simulink library "aerolibatmos2"  (Simulink 5.0)
values from neighbouring files (symbols this model uses):
  s = aeroliblist    [asbhelp.m]
undefined symbols (not defined in the file or in its folder): HDBK, kg, m, MIL, STD
libraries: aerolibconvert x7, aerolibatmos2 x3
settings Model: Creator=sgage  LastModifiedBy=sgage  ExtModeAutoUpdateStatusClock=off

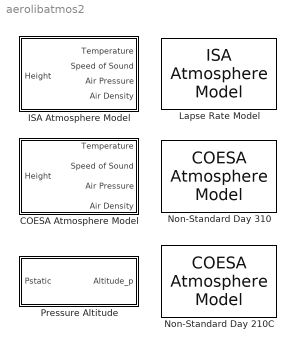
== system aerolibatmos2 ==
  COESA Atmosphere Model : Subsystem  mask(Atmosphere Model){units=Metric (MKS), spec=1976 COESA-extended U.S. Standard Atmosphere, model=Profile, profile_var=High temperature, profile_percent=1%, profile_alt=5 km (16404 ft), envelope_var=High temperature, envelope_percent=1%, action=Warning}
      mask prompts: spec "Specification:"; model "Atmospheric model type:"; profile_var "Extreme parameter:"; profile_percent "Frequency of occurrence:"; profile_alt "Altitude of extreme value:"; envelope_var "Extreme parameter:"; envelope_percent "Frequency of occurrence:"; action "Action for out of range input:"
      mask help:
      | Calculate various atmosphere models including 1976 COESA-extended U.S. Standard Atmosphere, MIL-HDBK-310, and MIL-STD-210C.  Given geopotential altitude, calculate absolute temperature, pressure and density using standard interpolation formulas.
      |
      | The COESA model extrapolates temperature linearly and pressure/density logarithmically beyond the range
      |
      | 	0 <= altitude <= 84852 meters (geopotential)
      |
      | The MIL specifications are not extrapolated beyond their defined altitudes which are typically
      |
      | 	0 <= altitude <= 80000 meters (geometric)
      |
      | Depending on the given information either density or pressure is calculated using a perfect gas relationship.
      |
      | The unit system selected applies to both input and outputs.
      mask init:
      | [ports] = aeroicon('aeroblkatmos','icon');
      | [x y miny txt] = aeroimage('atmosphere');
      mask Help: web(asbhelp('COESA Atmosphere Model'));
      mask StyleString: popup(Metric (MKS)|English (Velocity in ft/s)|English (Velocity in kts)),popup(1976 COESA-extended U.S. Standard Atmosphere|MIL-HDBK-310|MIL-STD-210C),popup(Profile|Envelope),popup(High temperature|Low temperature|High density|Low density),popup(1%|10%),popup(5 km (16404 ft)|10 km (32808 ft)|20 km (65617 ft)|30 km (98425 ft)|40 km (131234 ft)),popup(High temperature|Low temperature|High density|Low density|High pressure|Low pressure),popup(Extreme values|1%|5%|10%|20%),popup(None|Warning|Error)
      mask CallbackString: aeroicon('aeroblkatmos');|aeroicon('aeroblkatmos');|aeroicon('aeroblkatmos');||||||
      mask Display:
      | port_label(ports(1).type,ports(1).port,ports(1).txt,'texmode','on');
      | port_label(ports(2).type,ports(2).port,ports(2).txt,'texmode','on');
      | port_label(ports(3).type,ports(3).port,ports(3).txt,'texmode','on');
      | port_label(ports(4).type,ports(4).port,ports(4).txt,'texmode','on');
      | port_label(ports(5).type,ports(5).port,ports(5).txt,'texmode','on');
      | plot(x,y)
      | text(0.5,miny-.07,txt,'HorizontalAlignment','center');
  ISA Atmosphere Model : Subsystem  mask(International Standard Atmosphere Model){custom=off, g=9.80665, gamma=1.4, R=287.0531, L=0.0065, h_trop=11000, h_strat=20000, rho0=1.225, P0=101325, T0=288.15}
      mask prompts: custom "Change atmospheric parameters"; g "Acceleration due to gravity (m/s^2):"; gamma "Ratio of specific heats:"; R "Characteristic gas constant (J/Kg/K):"; L "Lapse rate (K/m):"; h_trop "Height of troposphere (m):"; h_strat "Height of tropopause (m):"; rho0 "Air density at mean sea level (Kg/m^3):"; P0 "Ambient pressure at mean sea level (N/m^2):"; T0 "Ambient temperature at mean sea level (K):"
      mask help:
      | Compute International Standard Atmosphere (ISA) model for altitudes between 0 Km and 20 Km using a lapse rate method.
      |
      | Select change atmospheric parameters to create custom atmosphere.
      mask init:
      | ports = aeroicon('aeroblkisa','icon');
      | [x y miny txt] = aeroimage('atmosphere');
      mask Help: web(asbhelp('isaatmospheremodel'));
      mask CallbackString: aeroicon('aeroblkisa')|||||||||
      mask Display:
      | port_label('input',1,'h (m)','texmode','on');
      | port_label('output',1,'T (K)','texmode','on');
      | port_label('output',2,'a (m/s)','texmode','on');
      | port_label('output',3,'P (Pa)','texmode','on');
      | port_label('output',4,'\rho (kg/m^3)','texmode','on');
      | plot(x,y)
      | text(0.5,miny-.07,txt,'HorizontalAlignment','center');
  Lapse Rate Model : aerolibatmos2/ISA Atmosphere Model  custom=on  g=9.80665  gamma=1.4  R=287.0531  L=0.0065  h_trop=11000  h_strat=20000  rho0=1.225  P0=101325  T0=288.15
  Non-Standard Day 210C : aerolibatmos2/COESA Atmosphere Model  units=Metric (MKS)  spec=MIL-STD-210C  model=Profile  profile_var=High temperature  profile_percent=1%  profile_alt=5 km (16404 ft)  envelope_var=High temperature  envelope_percent=1%  action=Warning
  Non-Standard Day 310 : aerolibatmos2/COESA Atmosphere Model  units=Metric (MKS)  spec=MIL-HDBK-310  model=Profile  profile_var=High temperature  profile_percent=1%  profile_alt=5 km (16404 ft)  envelope_var=High temperature  envelope_percent=1%  action=Warning
  Pressure Altitude : Subsystem  mask(Pressure Altitude){units=Metric (MKS), action=Warning}
      mask prompts: action "Action for out of range input:"
      mask help:
      | Calculate pressure altitude based on ambient pressure.
      |
      | Pressure altitude is the altitude in the 1976 COESA-extended U.S. Standard Atmosphere with specified ambient pressure.  Pressure altitude is also known as the mean sea level altitude (MSL).
      mask init:
      | ports = aeroicon('aeroblkpalt','icon');
      mask Help: web(asbhelp('pressurealtitude'));
      mask StyleString: popup(Metric (MKS)|English),popup(None|Warning|Error)
      mask Display:
      | port_label(ports(1).type,ports(1).port,ports(1).txt,'texmode','on');
      | port_label(ports(2).type,ports(2).port,ports(2).txt,'texmode','on');

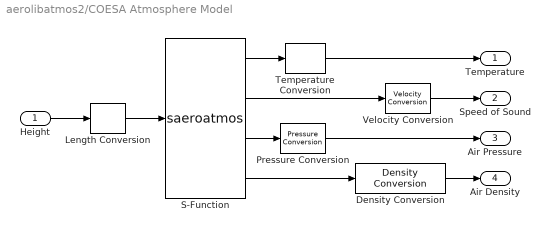
== system aerolibatmos2/COESA Atmosphere Model ==
  Height : Inport
  Density Conversion : aerolibconvert/Density Conversion  IU=kg/m^3  OU=kg/m^3
  Length Conversion : aerolibconvert/Length Conversion  IU=m  OU=m
  Pressure Conversion : aerolibconvert/Pressure Conversion  IU=Pa  OU=Pa
  S-Function : S-Function  FunctionName=saeroatmos  Parameters=spec,model,profile_var,profile_percent,profile_alt,envelope_var,envelope_percent,action  SFunctionModules=aeroatmcoesa aeroatmenvelope310 aeroatmenvelope210c aeroatmprofile310 aeroatmprofile210c
  Temperature Conversion : aerolibconvert/Temperature Conversion  IU=K  OU=K
  Velocity Conversion : aerolibconvert/Velocity Conversion  IU=m/s  OU=m/s
  Temperature : Outport
  Speed of Sound : Outport  Port=2
  Air Pressure : Outport  Port=3
  Air Density : Outport  Port=4
  wires:
  Length Conversion/1 -> S-Function/1
  Velocity Conversion/1 -> Speed of Sound/1
  S-Function/2 -> Velocity Conversion/1
  S-Function/1 -> Temperature Conversion/1
  S-Function/3 -> Pressure Conversion/1
  S-Function/4 -> Density Conversion/1
  Temperature Conversion/1 -> Temperature/1
  Height/1 -> Length Conversion/1
  Pressure Conversion/1 -> Air Pressure/1
  Density Conversion/1 -> Air Density/1

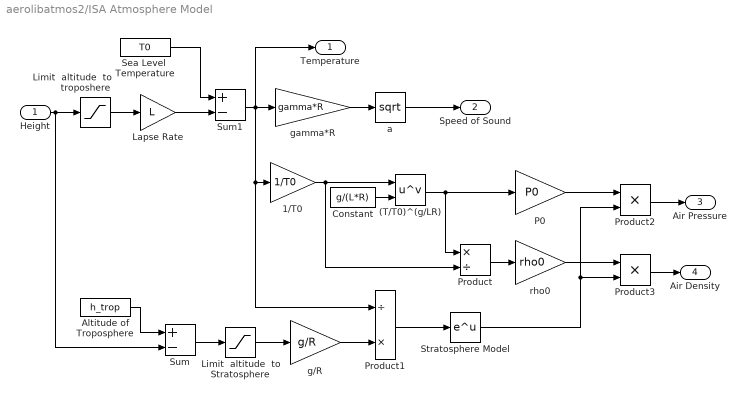
== system aerolibatmos2/ISA Atmosphere Model ==
  Height : Inport
  "(T/T0)^(g/LR) " : Math  Operator=pow
  1/T0 : Gain  Gain=1/T0  SaturateOnIntegerOverflow=on
  Altitude of Troposphere : Constant  Value=h_trop  ShowAdditionalParam=on
  Constant : Constant  Value=g/(L*R)  ShowAdditionalParam=on
  Lapse Rate : Gain  Gain=L  SaturateOnIntegerOverflow=on
  Limit  altitude  to Stratosphere : Saturate  UpperLimit=0  LowerLimit=h_trop-h_strat
  Limit  altitude  to troposhere : Saturate  UpperLimit=h_trop  LowerLimit=0
  P0 : Gain  Gain=P0  SaturateOnIntegerOverflow=on
  Product : Product  Inputs=*/  SaturateOnIntegerOverflow=on  InputSameDT=on
  Product1 : Product  Inputs=/*  SaturateOnIntegerOverflow=on  InputSameDT=on
  Product2 : Product  SaturateOnIntegerOverflow=on  InputSameDT=on
  Product3 : Product  SaturateOnIntegerOverflow=on  InputSameDT=on
  Sea Level  Temperature : Constant  Value=T0  ShowAdditionalParam=on
  Stratosphere Model : Math
  Sum : Sum  Inputs=+-  SaturateOnIntegerOverflow=on  InputSameDT=on
  Sum1 : Sum  Inputs=+-  SaturateOnIntegerOverflow=on  InputSameDT=on
  a : Math  Operator=sqrt
  g/R : Gain  Gain=g/R  SaturateOnIntegerOverflow=on
  gamma*R : Gain  Gain=gamma*R  SaturateOnIntegerOverflow=on
  rho0 : Gain  Gain=rho0  SaturateOnIntegerOverflow=on
  Temperature : Outport
  Speed of Sound : Outport  Port=2
  Air Pressure : Outport  Port=3
  Air Density : Outport  Port=4
  wires:
  Limit  altitude  to Stratosphere/1 -> g/R/1
  Sum/1 -> Limit  altitude  to Stratosphere/1
  Altitude of Troposphere/1 -> Sum/1
  Product1/1 -> Stratosphere Model/1
  g/R/1 -> Product1/2
  Stratosphere Model/1 -> Product3/2, Product2/2
  Product3/1 -> Air Density/1
  rho0/1 -> Product3/1
  Product2/1 -> Air Pressure/1
  P0/1 -> Product2/1
  Sea Level  Temperature/1 -> Sum1/1
  Lapse Rate/1 -> Sum1/2
  Sum1/1 -> Product1/1, 1/T0/1, gamma*R/1, Temperature/1
  a/1 -> Speed of Sound/1
  gamma*R/1 -> a/1
  1/T0/1 -> Product/2, "(T/T0)^(g/LR) "/1
  "(T/T0)^(g/LR) "/1 -> P0/1, Product/1
  Product/1 -> rho0/1
  Limit  altitude  to troposhere/1 -> Lapse Rate/1
  Height/1 -> Sum/2, Limit  altitude  to troposhere/1
  Constant/1 -> "(T/T0)^(g/LR) "/2

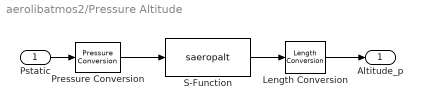
== system aerolibatmos2/Pressure Altitude ==
  Pstatic : Inport
  Length Conversion : aerolibconvert/Length Conversion  IU=m  OU=m
  Pressure Conversion : aerolibconvert/Pressure Conversion  IU=Pa  OU=Pa
  S-Function : S-Function  FunctionName=saeropalt  Parameters=action  SFunctionModules=aeroatmcoesa
  Altitude_p : Outport
  wires:
  Pressure Conversion/1 -> S-Function/1
  Length Conversion/1 -> Altitude_p/1
  Pstatic/1 -> Pressure Conversion/1
  S-Function/1 -> Length Conversion/1
